simulink model "Galvanometro"  (Simulink 7.1)
settings: Solver=ode45  StartTime=0.0  StopTime=10.0  RelTol=1e-3
settings Model: Creator=George  LastModifiedBy=George

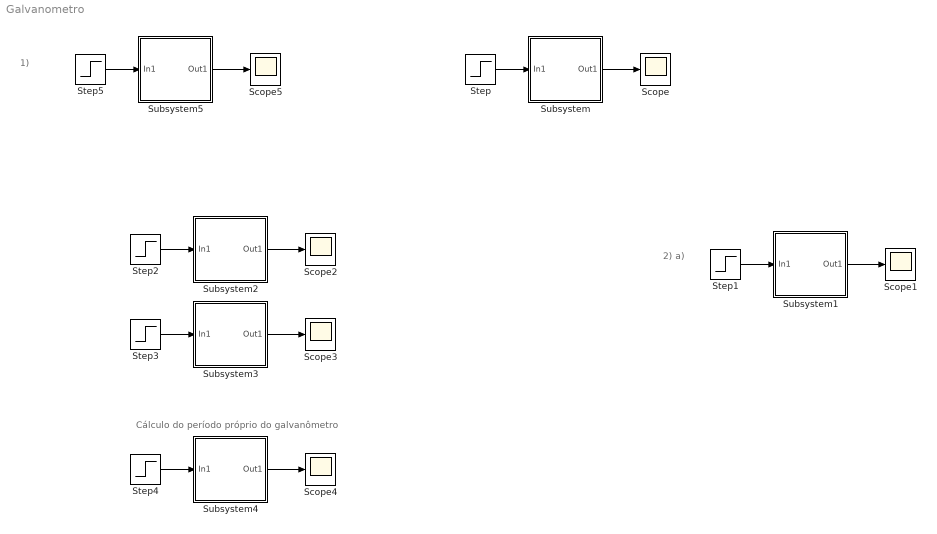
== system Galvanometro ==
  note: Cálculo do período próprio do galvanômetro
  note: 1)
  note: 2) a)
  Scope{,1..5} (6 alike) : Scope
      Scope2 settings: SaveName=ScopeData2
      Scope3 settings: SaveName=ScopeData3
      Scope4 settings: SaveName=ScopeData4
      Scope5 settings: SaveName=ScopeData5
  Step{,1..3,5} (5 alike) : Step  Time=0  After=9  SampleTime=0
  Step4 : Step  Time=0  After=0  SampleTime=0
  Subsystem : Subsystem  mask{J=0.5, B=0, phi=5, rg=1, R=49, K=4}
      mask Display: disp('Galvanometro')
  Subsystem1 : Subsystem  mask{J=0.5, B=0, phi=10, rg=1, R=34.35, K=4}
      mask Display: disp('Galvanometro')
  Subsystem2 : Subsystem  mask{J=0.5, B=0, phi=20, rg=1, R=49, K=4}
      mask Display: disp('Galvanometro')
  Subsystem3 : Subsystem  mask{J=0.5, B=0, phi=20, rg=1, R=49, K=4}
      mask Display: disp('Galvanometro')
  Subsystem4 : Subsystem  mask{J=0.5, B=0.5, phi=0, rg=1, R=49, K=4}
      mask Display: disp('Galvanometro')
  Subsystem5 : Subsystem  mask{J=0.5, B=0, phi=10, rg=1, R=49, K=4}
      mask Display: disp('Galvanometro')
  wires:
  Step/1 -> Subsystem/1(In1)
  Subsystem/1(Out1) -> Scope/1
  Step1/1 -> Subsystem1/1(In1)
  Subsystem1/1(Out1) -> Scope1/1
  Step2/1 -> Subsystem2/1(In1)
  Subsystem2/1(Out1) -> Scope2/1
  Step3/1 -> Subsystem3/1(In1)
  Subsystem3/1(Out1) -> Scope3/1
  Step4/1 -> Subsystem4/1(In1)
  Subsystem4/1(Out1) -> Scope4/1
  Step5/1 -> Subsystem5/1(In1)
  Subsystem5/1(Out1) -> Scope5/1

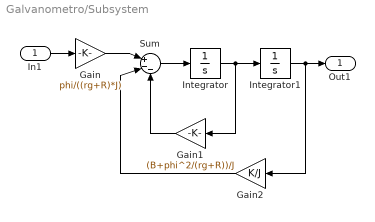
== system Galvanometro/Subsystem ==
  In1 : Inport
  Gain : Gain  Gain=phi/((rg+R)*J)  ParameterDataType=sfix(16)  ParameterScaling=2^0  OutDataType=sfix(16)  OutScaling=2^0
  Gain1 : Gain  Orientation=left  Gain=(B+phi^2/(rg+R))/J  ParameterDataType=sfix(16)  ParameterScaling=2^0  OutDataType=sfix(16)  OutScaling=2^0
  Gain2 : Gain  Orientation=left  Gain=K/J  ParameterDataType=sfix(16)  ParameterScaling=2^0  OutDataType=sfix(16)  OutScaling=2^0
  Integrator : Integrator
  Integrator1 : Integrator
  Sum : Sum  Inputs=|+--  OutDataType=sfix(16)  OutScaling=2^0
  Out1 : Outport
  wires:
  Sum/1 -> Integrator/1
  Integrator/1 -> Integrator1/1, Gain1/1
  Gain1/1 -> Sum/3
  Integrator1/1 -> Gain2/1, Out1/1
  Gain2/1 -> Sum/2
  In1/1 -> Gain/1
  Gain/1 -> Sum/1

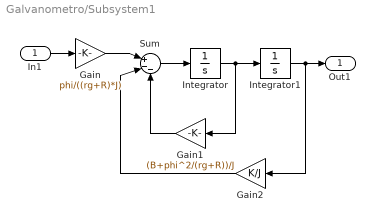
== system Galvanometro/Subsystem1 ==
  In1 : Inport
  Gain : Gain  Gain=phi/((rg+R)*J)  ParameterDataType=sfix(16)  ParameterScaling=2^0  OutDataType=sfix(16)  OutScaling=2^0
  Gain1 : Gain  Orientation=left  Gain=(B+phi^2/(rg+R))/J  ParameterDataType=sfix(16)  ParameterScaling=2^0  OutDataType=sfix(16)  OutScaling=2^0
  Gain2 : Gain  Orientation=left  Gain=K/J  ParameterDataType=sfix(16)  ParameterScaling=2^0  OutDataType=sfix(16)  OutScaling=2^0
  Integrator : Integrator
  Integrator1 : Integrator
  Sum : Sum  Inputs=|+--  OutDataType=sfix(16)  OutScaling=2^0
  Out1 : Outport
  wires:
  Sum/1 -> Integrator/1
  Integrator/1 -> Integrator1/1, Gain1/1
  Gain1/1 -> Sum/3
  Integrator1/1 -> Gain2/1, Out1/1
  Gain2/1 -> Sum/2
  In1/1 -> Gain/1
  Gain/1 -> Sum/1

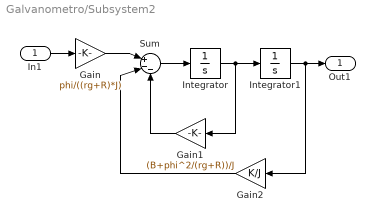
== system Galvanometro/Subsystem2 ==
  In1 : Inport
  Gain : Gain  Gain=phi/((rg+R)*J)  ParameterDataType=sfix(16)  ParameterScaling=2^0  OutDataType=sfix(16)  OutScaling=2^0
  Gain1 : Gain  Orientation=left  Gain=(B+phi^2/(rg+R))/J  ParameterDataType=sfix(16)  ParameterScaling=2^0  OutDataType=sfix(16)  OutScaling=2^0
  Gain2 : Gain  Orientation=left  Gain=K/J  ParameterDataType=sfix(16)  ParameterScaling=2^0  OutDataType=sfix(16)  OutScaling=2^0
  Integrator : Integrator
  Integrator1 : Integrator
  Sum : Sum  Inputs=|+--  OutDataType=sfix(16)  OutScaling=2^0
  Out1 : Outport
  wires:
  Sum/1 -> Integrator/1
  Integrator/1 -> Integrator1/1, Gain1/1
  Gain1/1 -> Sum/3
  Integrator1/1 -> Gain2/1, Out1/1
  Gain2/1 -> Sum/2
  In1/1 -> Gain/1
  Gain/1 -> Sum/1

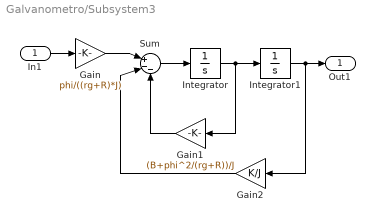
== system Galvanometro/Subsystem3 ==
  In1 : Inport
  Gain : Gain  Gain=phi/((rg+R)*J)  ParameterDataType=sfix(16)  ParameterScaling=2^0  OutDataType=sfix(16)  OutScaling=2^0
  Gain1 : Gain  Orientation=left  Gain=(B+phi^2/(rg+R))/J  ParameterDataType=sfix(16)  ParameterScaling=2^0  OutDataType=sfix(16)  OutScaling=2^0
  Gain2 : Gain  Orientation=left  Gain=K/J  ParameterDataType=sfix(16)  ParameterScaling=2^0  OutDataType=sfix(16)  OutScaling=2^0
  Integrator : Integrator
  Integrator1 : Integrator
  Sum : Sum  Inputs=|+--  OutDataType=sfix(16)  OutScaling=2^0
  Out1 : Outport
  wires:
  Sum/1 -> Integrator/1
  Integrator/1 -> Integrator1/1, Gain1/1
  Gain1/1 -> Sum/3
  Integrator1/1 -> Gain2/1, Out1/1
  Gain2/1 -> Sum/2
  In1/1 -> Gain/1
  Gain/1 -> Sum/1

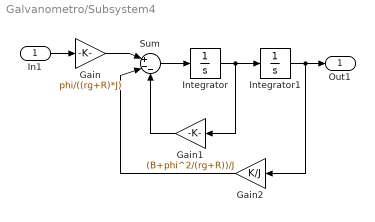
== system Galvanometro/Subsystem4 ==
  In1 : Inport
  Gain : Gain  Gain=phi/((rg+R)*J)  ParameterDataType=sfix(16)  ParameterScaling=2^0  OutDataType=sfix(16)  OutScaling=2^0
  Gain1 : Gain  Orientation=left  Gain=(B+phi^2/(rg+R))/J  ParameterDataType=sfix(16)  ParameterScaling=2^0  OutDataType=sfix(16)  OutScaling=2^0
  Gain2 : Gain  Orientation=left  Gain=K/J  ParameterDataType=sfix(16)  ParameterScaling=2^0  OutDataType=sfix(16)  OutScaling=2^0
  Integrator : Integrator
  Integrator1 : Integrator  InitialCondition=pi/3
  Sum : Sum  Inputs=|+--  OutDataType=sfix(16)  OutScaling=2^0
  Out1 : Outport
  wires:
  Sum/1 -> Integrator/1
  Integrator/1 -> Integrator1/1, Gain1/1
  Gain1/1 -> Sum/3
  Integrator1/1 -> Gain2/1, Out1/1
  Gain2/1 -> Sum/2
  In1/1 -> Gain/1
  Gain/1 -> Sum/1

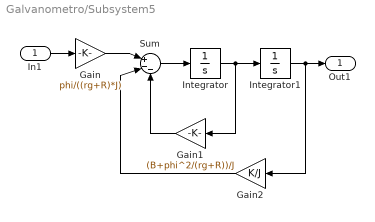
== system Galvanometro/Subsystem5 ==
  In1 : Inport
  Gain : Gain  Gain=phi/((rg+R)*J)  ParameterDataType=sfix(16)  ParameterScaling=2^0  OutDataType=sfix(16)  OutScaling=2^0
  Gain1 : Gain  Orientation=left  Gain=(B+phi^2/(rg+R))/J  ParameterDataType=sfix(16)  ParameterScaling=2^0  OutDataType=sfix(16)  OutScaling=2^0
  Gain2 : Gain  Orientation=left  Gain=K/J  ParameterDataType=sfix(16)  ParameterScaling=2^0  OutDataType=sfix(16)  OutScaling=2^0
  Integrator : Integrator
  Integrator1 : Integrator
  Sum : Sum  Inputs=|+--  OutDataType=sfix(16)  OutScaling=2^0
  Out1 : Outport
  wires:
  Sum/1 -> Integrator/1
  Integrator/1 -> Integrator1/1, Gain1/1
  Gain1/1 -> Sum/3
  Integrator1/1 -> Gain2/1, Out1/1
  Gain2/1 -> Sum/2
  In1/1 -> Gain/1
  Gain/1 -> Sum/1
